simulink model "holo"  (R2012b)
settings: Solver=FixedStepDiscrete  SolverMode=SingleTasking  StartTime=0.0  StopTime=160000  RelTol=1e-3
undefined symbols (not defined in the file): xlipgetpartsetting
libraries: xbsIndex_r4 x3259, casper_library_misc x36, simulink x18, dspsigops x12, casper_library_delays x8, xps_library x5, casper_library_multipliers x4
(part 1 of 34)
settings Model: Creator=Administrator  LastModifiedBy=brains
settings DataIOCC: SignalLoggingSaveFormat=ModelDataLogs
settings OptimizationCC: InitFltsAndDblsToZero=on
settings DebuggingCC: FcnCallInpInsideContextMsg=UseLocalSettings  StrictBusMsg=Warning
settings GRTTargetCC: CombineOutputUpdateFcns=off  GRTInterface=on

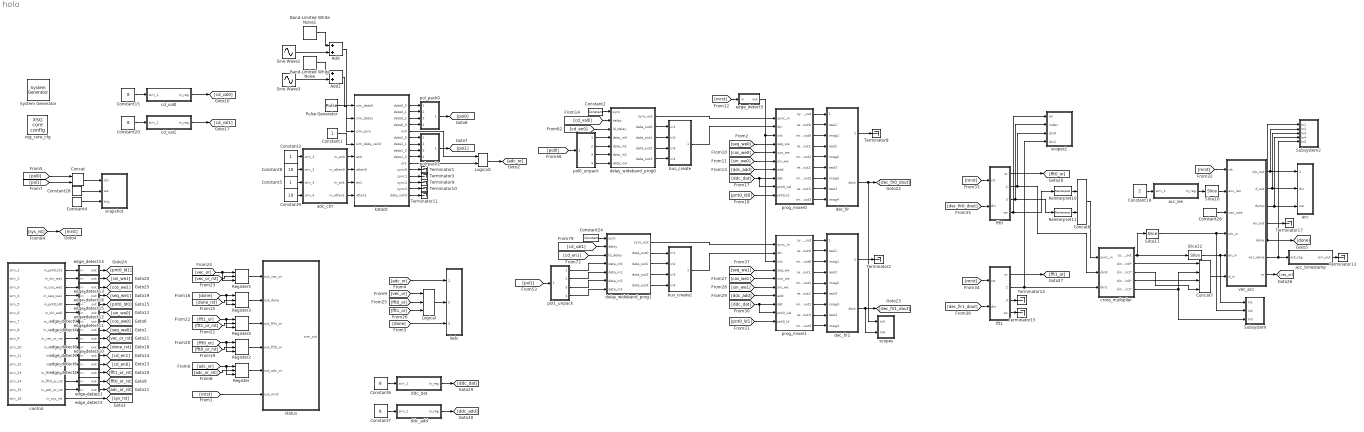
== system holo ==
  " System Generator" : xbsIndex_r4/ System Generator  Tag=genX  xilinxfamily=virtex5  part=xc5vsx95t  speed=-1  package=ff1136  synthesis_tool=XST  clock_wrapper=Clock Enables  directory=./holo/sysgen  proj_type=Project Navigator  Synth_file=XST Defaults  Impl_file=ISE Defaults  testbench=off  simulink_period=1  sysclk_period=5  dcm_input_clock_period=100  incr_netlist=off  trim_vbits=Everywhere in SubSystem  dbl_ovrd=According to Block Masks  core_generation=According to Block Masks  run_coregen=off  deprecated_control=off  eval_field=0  block_type=sysgen
      settings: block_version=10.1.3
  Add : Sum
  Add1 : Sum
  Band-Limited White Noise : simulink/Sources/Band-Limited White Noise  Cov=[0.02]  Ts=0.1  seed=[23341]
  Band-Limited White Noise1 : simulink/Sources/Band-Limited White Noise  Cov=[0.01]  Ts=0.1  seed=[23345]
  Concat : xbsIndex_r4/Concat  num_inputs=2  dbl_ovrd=off  block_type=concat
      settings: block_version=10.1.3
  Concat7 : xbsIndex_r4/Concat  num_inputs=4  dbl_ovrd=off  block_type=concat
      settings: block_version=10.1.3
  Concat8 : xbsIndex_r4/Concat  num_inputs=2  dbl_ovrd=off  block_type=concat
      settings: block_version=10.1.3
  Constant1 : Constant  SampleTime=1/4
  Constant{6..7,15,20} (4 alike) : Constant  Value=8
  Constant19 : Constant  Value=2
  Constant2 : xbsIndex_r4/Constant  const=0  gui_display_data_type=Fixed-point  arith_type=Boolean  n_bits=16  bin_pt=14  preci_type=Single  exp_width=8  frac_width=24  explicit_period=on  period=1  equ=P=C  opselect=C  inp2=PCIN>>17  opr=+  inp1=P  carry=CIN  dbl_ovrd=off  block_type=constant
  Constant24 : xbsIndex_r4/Constant  const=0  gui_display_data_type=Fixed-point  arith_type=Boolean  n_bits=16  bin_pt=14  preci_type=Single  exp_width=8  frac_width=24  explicit_period=on  period=1  equ=P=C  opselect=C  inp2=PCIN>>17  opr=+  inp1=P  carry=CIN  dbl_ovrd=off  block_type=constant
  Constant26 : xbsIndex_r4/Constant  const=4096  gui_display_data_type=Fixed-point  arith_type=Unsigned  n_bits=13  bin_pt=0  preci_type=Single  exp_width=8  frac_width=24  explicit_period=off  period=1  equ=P=C  opselect=C  inp2=PCIN>>17  opr=+  inp1=P  carry=CIN  dbl_ovrd=off  block_type=constant
  Constant28 : xbsIndex_r4/Constant  const=1  gui_display_data_type=Fixed-point  arith_type=Boolean  n_bits=16  bin_pt=14  preci_type=Single  exp_width=8  frac_width=24  explicit_period=off  period=1  equ=P=C  opselect=C  inp2=PCIN>>17  opr=+  inp1=P  carry=CIN  dbl_ovrd=off  block_type=constant
  Constant3 : Constant
  Constant4 : xbsIndex_r4/Constant  const=1  gui_display_data_type=Fixed-point  arith_type=Boolean  n_bits=16  bin_pt=14  preci_type=Single  exp_width=8  frac_width=24  explicit_period=off  period=1  equ=P=C  opselect=C  inp2=PCIN>>17  opr=+  inp1=P  carry=CIN  dbl_ovrd=off  block_type=constant
  Constant5 : Constant
  Constant8 : Constant  Value=10
  Constant9 : Constant  Value=10
  Logical : xbsIndex_r4/Logical  logical_function=OR  inputs=3  en=off  latency=1  precision=Full  arith_type=Unsigned  n_bits=16  bin_pt=0  align_bp=on  dbl_ovrd=off  block_type=logical
  Logical1 : xbsIndex_r4/Logical  logical_function=OR  inputs=2  en=off  latency=1  precision=Full  arith_type=Unsigned  n_bits=16  bin_pt=0  align_bp=on  dbl_ovrd=off  block_type=logical
  Pulse Generator : DiscretePulseGenerator  Period=2^14  PhaseDelay=11  SampleTime=1/4
  Register{,2..5} (5 alike) : xbsIndex_r4/Register  init=0  rst=on  en=on  dbl_ovrd=off  block_type=register
  Reinterpret10 : xbsIndex_r4/Reinterpret  force_arith_type=on  arith_type=Unsigned  force_bin_pt=on  bin_pt=0  block_type=reinterpret
      settings: infoedit="Changes signal type without altering the binary representation.   You can changed the signal between signed and unsigned, and relocate the binary point.<br><br>Hardware notes: In hardware this block costs nothing.<br><br>Example:  Suppose the input is 6 bits wide, signed, with 2 fractional bits, and the output is forced to unsigned with 0 fractional bits.  Then an input of -2.0 (1110.00 in binary 2's complement) becomes an output of 56 (111000 in binary)."
  Reinterpret11 : xbsIndex_r4/Reinterpret  force_arith_type=on  arith_type=Unsigned  force_bin_pt=on  bin_pt=0  block_type=reinterpret
      settings: infoedit="Changes signal type without altering the binary representation.   You can changed the signal between signed and unsigned, and relocate the binary point.<br><br>Hardware notes: In hardware this block costs nothing.<br><br>Example:  Suppose the input is 6 bits wide, signed, with 2 fractional bits, and the output is forced to unsigned with 0 fractional bits.  Then an input of -2.0 (1110.00 in binary 2's complement) becomes an output of 56 (111000 in binary)."
  Sine Wave2 : Sin  Amplitude=0.1  Frequency=57.5/524 * 2 * pi *4  Samples=57.5/524  SampleTime=1/4
  Sine Wave3 : Sin  Amplitude=0.2  Frequency=57.5/524 * 2 * pi *4  Samples=57.5/524  SampleTime=1/4
  Slice10 : xbsIndex_r4/Slice  nbits=16  boolean_output=off  mode=Lower Bit Location + Width  bit1=0  base1=MSB of Input  bit0=0  base0=LSB of Input  dbl_ovrd=off  block_type=slice
      settings: infoedit="Extracts a given range of bits from each input sample and presents it at the output.  The output type is ordinarily unsigned with binary point at zero, but can be Boolean when the slice is one bit wide.<P><P>Hardware notes: In hardware this block costs nothing."  block_version=10.1.3
  Slice11 : xbsIndex_r4/Slice  nbits=12  boolean_output=off  mode=Lower Bit Location + Width  bit1=0  base1=MSB of Input  bit0=0  base0=LSB of Input  dbl_ovrd=off  block_type=slice
      settings: block_version=10.1.3
  Slice12 : xbsIndex_r4/Slice  nbits=1  boolean_output=on  mode=Upper Bit Location + Width  bit1=0  base1=MSB of Input  bit0=0  base0=LSB of Input  dbl_ovrd=off  block_type=slice
      settings: infoedit="Extracts a given range of bits from each input sample and presents it at the output.  The output type is ordinarily unsigned with binary point at zero, but can be Boolean when the slice is one bit wide.<P><P>Hardware notes: In hardware this block costs nothing."  block_version=10.1.3
  Subsystem : Subsystem
  Subsystem2 : Subsystem
  Terminator{1..3,8..11,13..15,17} (11 alike) : Terminator
  acc : Subsystem  mask{bit_width=76, bit_width_o=32, num_chans=12}
      mask prompts: bit_width "Bit width in"; bit_width_o "Bit width out"; num_chans "Number of channels (2^?)"
  acc_len : Subsystem  Tag=xps:sw_reg  AncestorBlock=xps_library/software register  mask(swreg){io_dir=From Processor, io_delay=0, sample_period=1, names=reg, bitwidths=32, bin_pts=0, arith_types=0, sim_port=on, show_format=on}
      mask prompts: io_dir "I/O direction"; io_delay "I/O delay"; sample_period "Sample period"; names "Bitfield names [msb...lsb]"; bitwidths "Bitfield widths"; bin_pts "Bitfield binary pts"; arith_types "Bitfield types, ufix=0, fix=1, bool=2"; sim_port "Provide sim input/output?"; show_format "Print format string?"
      mask help: A 32-bit software-accessible register. Can be divided into bitfields of varying widths and types using the fields in the block mask.
      mask init:
      | swreg_init(gcb)
      settings: AttributesFormatString=1input:uf32.0
      mask TypeOptions io_dir: To Processor | From Processor
      mask Callback io_dir:
      | mask_enables = get_param(gcb, 'MaskEnables');
      | mask_names = get_param(gcb, 'MaskNames');
      | if strcmp(get_param(gcb, 'io_dir'), 'To Processor'),
      |     mask_enables{ismember(mask_names, 'sample_period')} = 'off';
      | else
      |     mask_enables{ismember(mask_names, 'sample_period')} = 'on';
      | end
      | set_param(gcb, 'MaskEnables', mask_enables);
  acc_timestamp : Subsystem  Tag=xps:sw_reg  AncestorBlock=xps_library/software register  mask(swreg){io_dir=To Processor, io_delay=0, sample_period=1, names=reg, bitwidths=32, bin_pts=0, arith_types=0, sim_port=on, show_format=on}
      mask prompts: io_dir "I/O direction"; io_delay "I/O delay"; sample_period "Sample period"; names "Bitfield names [msb...lsb]"; bitwidths "Bitfield widths"; bin_pts "Bitfield binary pts"; arith_types "Bitfield types, ufix=0, fix=1, bool=2"; sim_port "Provide sim input/output?"; show_format "Print format string?"
      mask help: A 32-bit software-accessible register. Can be divided into bitfields of varying widths and types using the fields in the block mask.
      mask init:
      | swreg_init(gcb)
      settings: AttributesFormatString=1output:uf32.0
      mask TypeOptions io_dir: To Processor | From Processor
      mask Callback io_dir:
      | mask_enables = get_param(gcb, 'MaskEnables');
      | mask_names = get_param(gcb, 'MaskNames');
      | if strcmp(get_param(gcb, 'io_dir'), 'To Processor'),
      |     mask_enables{ismember(mask_names, 'sample_period')} = 'off';
      | else
      |     mask_enables{ismember(mask_names, 'sample_period')} = 'on';
      | end
      | set_param(gcb, 'MaskEnables', mask_enables);
  adc_ctrl : Subsystem  Tag=xps:sw_reg  AncestorBlock=xps_library/software register  DataTypeOverride=Double  MinMaxOverflowLogging=ForceOff  mask(swreg){io_dir=From Processor, io_delay=0, sample_period=1, names=[en0 atten0 en1 atten1], bitwidths=[1 6 1 6], bin_pts=[0 0 0 0], arith_types=[2 0 2 0], sim_port=on, show_format=on}
      mask prompts: io_dir "I/O direction"; io_delay "I/O delay"; sample_period "Sample period"; names "Bitfield names [msb...lsb]"; bitwidths "Bitfield widths"; bin_pts "Bitfield binary pts"; arith_types "Bitfield types, ufix=0, fix=1, bool=2"; sim_port "Provide sim input/output?"; show_format "Print format string?"
      mask help: A 32-bit software-accessible register. Can be divided into bitfields of varying widths and types using the fields in the block mask.
      mask init:
      | swreg_init(gcb)
      settings: AttributesFormatString=4 inputs:b,uf6.0,b,uf6.0
      mask TypeOptions io_dir: To Processor | From Processor
      mask Callback io_dir:
      | mask_enables = get_param(gcb, 'MaskEnables');
      | mask_names = get_param(gcb, 'MaskNames');
      | if strcmp(get_param(gcb, 'io_dir'), 'To Processor'),
      |     mask_enables{ismember(mask_names, 'sample_period')} = 'off';
      | else
      |     mask_enables{ismember(mask_names, 'sample_period')} = 'on';
      | end
      | set_param(gcb, 'MaskEnables', mask_enables);
  bus_create : Subsystem  AncestorBlock=casper_library_flow_control/bus_create  mask(bus_create){inputNum=4}
      mask prompts: inputNum "Number of inputs:"
      mask init:
      | bus_create_init(gcb,...
      |     'inputNum', inputNum);
  bus_create1 : Subsystem  AncestorBlock=casper_library_flow_control/bus_create  mask(bus_create){inputNum=4}
      mask prompts: inputNum "Number of inputs:"
      mask init:
      | bus_create_init(gcb,...
      |     'inputNum', inputNum);
  cd_val0 : Subsystem  Tag=xps:sw_reg  AncestorBlock=xps_library/software register  mask(swreg){io_dir=From Processor, io_delay=0, sample_period=1, names=reg, bitwidths=8, bin_pts=0, arith_types=0, sim_port=on, show_format=on}
      mask prompts: io_dir "I/O direction"; io_delay "I/O delay"; sample_period "Sample period"; names "Bitfield names [msb...lsb]"; bitwidths "Bitfield widths"; bin_pts "Bitfield binary pts"; arith_types "Bitfield types, ufix=0, fix=1, bool=2"; sim_port "Provide sim input/output?"; show_format "Print format string?"
      mask help: A 32-bit software-accessible register. Can be divided into bitfields of varying widths and types using the fields in the block mask.
      mask init:
      | swreg_init(gcb)
      settings: AttributesFormatString=1input:uf8.0
      mask TypeOptions io_dir: To Processor | From Processor
      mask Callback io_dir:
      | mask_enables = get_param(gcb, 'MaskEnables');
      | mask_names = get_param(gcb, 'MaskNames');
      | if strcmp(get_param(gcb, 'io_dir'), 'To Processor'),
      |     mask_enables{ismember(mask_names, 'sample_period')} = 'off';
      | else
      |     mask_enables{ismember(mask_names, 'sample_period')} = 'on';
      | end
      | set_param(gcb, 'MaskEnables', mask_enables);
  cd_val1 : Subsystem  Tag=xps:sw_reg  AncestorBlock=xps_library/software register  mask(swreg){io_dir=From Processor, io_delay=0, sample_period=1, names=reg, bitwidths=8, bin_pts=0, arith_types=0, sim_port=on, show_format=on}
      mask prompts: io_dir "I/O direction"; io_delay "I/O delay"; sample_period "Sample period"; names "Bitfield names [msb...lsb]"; bitwidths "Bitfield widths"; bin_pts "Bitfield binary pts"; arith_types "Bitfield types, ufix=0, fix=1, bool=2"; sim_port "Provide sim input/output?"; show_format "Print format string?"
      mask help: A 32-bit software-accessible register. Can be divided into bitfields of varying widths and types using the fields in the block mask.
      mask init:
      | swreg_init(gcb)
      settings: AttributesFormatString=1input:uf8.0
      mask TypeOptions io_dir: To Processor | From Processor
      mask Callback io_dir:
      | mask_enables = get_param(gcb, 'MaskEnables');
      | mask_names = get_param(gcb, 'MaskNames');
      | if strcmp(get_param(gcb, 'io_dir'), 'To Processor'),
      |     mask_enables{ismember(mask_names, 'sample_period')} = 'off';
      | else
      |     mask_enables{ismember(mask_names, 'sample_period')} = 'on';
      | end
      | set_param(gcb, 'MaskEnables', mask_enables);
  control : Subsystem  Tag=xps:sw_reg  AncestorBlock=xps_library/software register  DataTypeOverride=Double  MinMaxOverflowLogging=ForceOff  mask(swreg){io_dir=From Processor, io_delay=0, sample_period=1, names=[pnt0_ld1 sin_we1 cos_we1 seq_we1 pnt0_ld0 sin_we0 cos_we0 seq_we0 vec_or_rst done_rst cd_en1 cd_en0 fft1_or_rst fft0_or_rst adc_or_rst sys_rst], bitwidths=[1 1 1 1 1 1 1 1 1 1 1 1 1 1 1 1], bin_pts=[0 0 0 0 0 0 0 0 0 0 0 0 0 0 0 0], arith_types=[2 2 2 2 2 2 2 2 2 2 2 2 2 2 2 2], sim_port=on, show_format=on}
      mask prompts: io_dir "I/O direction"; io_delay "I/O delay"; sample_period "Sample period"; names "Bitfield names [msb...lsb]"; bitwidths "Bitfield widths"; bin_pts "Bitfield binary pts"; arith_types "Bitfield types, ufix=0, fix=1, bool=2"; sim_port "Provide sim input/output?"; show_format "Print format string?"
      mask help: A 32-bit software-accessible register. Can be divided into bitfields of varying widths and types using the fields in the block mask.
      mask init:
      | swreg_init(gcb)
      settings: AttributesFormatString=16 inputs:b,b,b,b,b,b,b,b,b,b,b,b,b,b,b,b
      mask TypeOptions io_dir: To Processor | From Processor
      mask Callback io_dir:
      | mask_enables = get_param(gcb, 'MaskEnables');
      | mask_names = get_param(gcb, 'MaskNames');
      | if strcmp(get_param(gcb, 'io_dir'), 'To Processor'),
      |     mask_enables{ismember(mask_names, 'sample_period')} = 'off';
      | else
      |     mask_enables{ismember(mask_names, 'sample_period')} = 'on';
      | end
      | set_param(gcb, 'MaskEnables', mask_enables);
  cross_multiplier : Subsystem  AncestorBlock=casper_library/Correlator/cross_multiplier  mask(cross_multiplier){streams=2, aggregation=1, bit_width_in=32, binary_point_in=18, bit_width_out=65, binary_point_out=36, mult_latency=3, add_latency=1, overflow=Saturate, quantisation=Round  (unbiased: even values), conv_latency=1}
      mask prompts: streams "Number input streams"; aggregation "Aggregation per stream"; bit_width_in "Bit width in"; binary_point_in "Binary point in"; bit_width_out "Bit width out"; binary_point_out "Binary point out"; mult_latency "Multiplier latency"; add_latency "Adder latency"; overflow "Overflow behaviour"; quantisation "Quantisation behaviour"; conv_latency "Bit width conversion latency"
      mask help: Cross multiplies aggregated complex input streams.
      mask init:
      | cross_multiplier_init(gcb, ...
      |     'streams', streams, ...
      |     'aggregation', aggregation, ...
      |     'bit_width_in', bit_width_in, ...
      |     'binary_point_in', binary_point_in, ...
      |     'bit_width_out', bit_width_out, ...
      |     'binary_point_out', binary_point_out, ...
      |     'mult_latency', mult_latency, ...
      |     'add_latency', add_latency, ...
      |     'overflow', overflow, ...
      |     'quantisation', quantisation, ...
      |     'conv_latency', conv_latency);
      mask TypeOptions overflow: Wrap | Saturate | Error
      mask TypeOptions quantisation: Truncate | Round  (unbiased: +/- Inf) | Round  (unbiased: even values)
  ddc_add : Subsystem  Tag=xps:sw_reg  AncestorBlock=xps_library/software register  DataTypeOverride=Double  MinMaxOverflowLogging=ForceOff  mask(swreg){io_dir=From Processor, io_delay=0, sample_period=1, names=reg, bitwidths=11, bin_pts=0, arith_types=0, sim_port=on, show_format=on}
      mask prompts: io_dir "I/O direction"; io_delay "I/O delay"; sample_period "Sample period"; names "Bitfield names [msb...lsb]"; bitwidths "Bitfield widths"; bin_pts "Bitfield binary pts"; arith_types "Bitfield types, ufix=0, fix=1, bool=2"; sim_port "Provide sim input/output?"; show_format "Print format string?"
      mask help: A 32-bit software-accessible register. Can be divided into bitfields of varying widths and types using the fields in the block mask.
      mask init:
      | swreg_init(gcb)
      settings: AttributesFormatString=1input:uf11.0
      mask TypeOptions io_dir: To Processor | From Processor
      mask Callback io_dir:
      | mask_enables = get_param(gcb, 'MaskEnables');
      | mask_names = get_param(gcb, 'MaskNames');
      | if strcmp(get_param(gcb, 'io_dir'), 'To Processor'),
      |     mask_enables{ismember(mask_names, 'sample_period')} = 'off';
      | else
      |     mask_enables{ismember(mask_names, 'sample_period')} = 'on';
      | end
      | set_param(gcb, 'MaskEnables', mask_enables);
  ddc_dat : Subsystem  Tag=xps:sw_reg  AncestorBlock=xps_library/software register  mask(swreg){io_dir=From Processor, io_delay=0, sample_period=1, names=reg, bitwidths=32, bin_pts=0, arith_types=0, sim_port=on, show_format=on}
      mask prompts: io_dir "I/O direction"; io_delay "I/O delay"; sample_period "Sample period"; names "Bitfield names [msb...lsb]"; bitwidths "Bitfield widths"; bin_pts "Bitfield binary pts"; arith_types "Bitfield types, ufix=0, fix=1, bool=2"; sim_port "Provide sim input/output?"; show_format "Print format string?"
      mask help: A 32-bit software-accessible register. Can be divided into bitfields of varying widths and types using the fields in the block mask.
      mask init:
      | swreg_init(gcb)
      settings: AttributesFormatString=1input:uf32.0
      mask TypeOptions io_dir: To Processor | From Processor
      mask Callback io_dir:
      | mask_enables = get_param(gcb, 'MaskEnables');
      | mask_names = get_param(gcb, 'MaskNames');
      | if strcmp(get_param(gcb, 'io_dir'), 'To Processor'),
      |     mask_enables{ismember(mask_names, 'sample_period')} = 'off';
      | else
      |     mask_enables{ismember(mask_names, 'sample_period')} = 'on';
      | end
      | set_param(gcb, 'MaskEnables', mask_enables);
  dec_fir : Subsystem  Tag=casper:dec_fir  AncestorBlock=casper_library_downconverter/dec_fir  mask(dec_fir){n_inputs=4, coeff=|, n_bits=25, n_bits_bp=24, quantization=Round  (unbiased: +/- Inf), add_latency=1, mult_latency=2, conv_latency=2, coeff_bit_width=18, coeff_bin_pt=17, absorb_adders=on, adder_imp=Behavioral, lshift=1}
      mask coeff=|
      | [-0.0447689124780572	0.00995075246871881	0.00901304692382896	0.00823242709364412	0.00758382054909261	0.00704464575825092	0.00659455775184286	0.00621523507993219	0.00589020244435913	0.00560468395514498	0.00534548245655601	0.00510088080992406	0.00486056141468576	0.00461554060398477	0.00435811487328397	0.00408181619532124	0.00378137394731173	0.00345268123054543	0.00309276360183094	0.00269974846331496	0.00227283357423222	0.00181225335677420	0.00131924186973398	0.000795991518688312	0.000245606760694299	-0.000327947755040654	-0.000919904991432013	-0.00152475948219077	-0.00213633748961542	-0.00274787324883546	-0.00335209103662813	-0.00394129266271928	-0.00450744985120910	-0.00504230086033329	-0.00553745058111782	-0.00598447326045595	-0.00637501691256493	-0.00670090841536199	-0.00695425823566635	-0.00712756368975998	-0.00721380962406963	-0.00720656539476785	-0.00710007703493642	-0.00688935352347128	-0.00657024611078542	-0.00613951971211587	-0.00559491544916114	-0.00493520350404395	-0.00416022554518398	-0.00327092609143079	-0.00226937229741241	-0.00115876176810638	5.65818574659195e-05	0.00137122567636325	0.00277865662797271	0.00427132277628112	0.00584068646574818	0.00747728890789533	0.00917082561895388	0.0109102319975610	0.0126837782072967	0.0144791724134059	0.0162836713178909	0.0180841968436693	0.0198674577379365	0.0216200747983420	0.0233287083740046	0.0249801867575000	0.0265616340642831	0.0280605961929114	0.0294651634730190	0.0307640886382082	0.0319468988075302	0.0330040002215846	0.0339267745567033	0.0347076657323696	0.0353402562318254	0.0358193320725324	0.0361409356903483	0.0363024061374426	0.0363024061374426	0.0361409356903483	0.0358193320725324	0.0353402562318254	0.0347076657323696	0.0339267745567033	0.0330040002215846	0.0319468988075302	0.0307640886382082	0.0294651634730190	0.0280605961929114	0.0265616340642831	0.0249801867575000	0.0233287083740046	0.0216200747983420	0.0198674577379365	0.0180841968436693	0.0162836713178909	0.0144791724134059	0.0126837782072967	0.0109102319975610	0.00917082561895388	0.00747728890789533	0.00584068646574818	0.00427132277628112	0.00277865662797271	0.00137122567636325	5.65818574659195e-05	-0.00115876176810638	-0.00226937229741241	-0.00327092609143079	-0.00416022554518398	-0.00493520350404395	-0.00559491544916114	-0.00613951971211587	-0.00657024611078542	-0.00688935352347128	-0.00710007703493642	-0.00720656539476785	-0.00721380962406963	-0.00712756368975998	-0.00695425823566635	-0.00670090841536199	-0.00637501691256493	-0.00598447326045595	-0.00553745058111782	-0.00504230086033329	-0.00450744985120910	-0.00394129266271928	-0.00335209103662813	-0.00274787324883546	-0.00213633748961542	-0.00152475948219077	-0.000919904991432013	-0.000327947755040654	0.000245606760694299	0.000795991518688312	0.00131924186973398	0.00181225335677420	0.00227283357423222	0.00269974846331496	0.00309276360183094	0.00345268123054543	0.00378137394731173	0.00408181619532124	0.00435811487328397	0.00461554060398477	0.00486056141468576	0.00510088080992406	0.00534548245655601	0.00560468395514498	0.00589020244435913	0.00621523507993219	0.00659455775184286	0.00704464575825092	0.00758382054909261	0.00823242709364412	0.00901304692382896	0.00995075246871881	-0.0447689124780572
      | ]
      mask prompts: n_inputs "Number of Parallel Streams"; coeff "Coefficients"; n_bits "Bit Width Out"; n_bits_bp "Bin Pt Out"; quantization "Quantization Behavior"; add_latency "Add Latency"; mult_latency "Mult Latency"; conv_latency "Convert latency"; coeff_bit_width "Coefficient bit width"; coeff_bin_pt "Coefficient binary point"; absorb_adders "Absorb adders into DSP slices"; adder_imp "Adder implementation"; lshift "Post adder-tree shift"
      mask help: FIR filter which can handle multiple time samples in parallel and decimates down to 1 time sample. If coefficients are symmetric, will automatically fold before multiplying.
      mask init:
      | dec_fir_init(gcb, ...
      |     'n_inputs', n_inputs, ...
      |     'coeff', coeff, ...
      |     'n_bits', n_bits, ...
      |     'n_bits_bp', n_bits_bp, ...
      |     'quantization', quantization, ...
      |     'add_latency', add_latency, ...
      |     'mult_latency', mult_latency, ...
      |     'conv_latency', conv_latency, ...
      |     'coeff_bit_width', coeff_bit_width, ...
      |     'coeff_bin_pt', coeff_bin_pt, ...
      |     'absorb_adders', absorb_adders, ...
      |     'adder_imp', adder_imp, ...
      |     'lshift', lshift);
      settings: AttributesFormatString=|
      | 160 taps
      | 25_24 r/i
      mask TypeOptions quantization: Truncate | Round  (unbiased: +/- Inf) | Round  (unbiased: Even Values)
      mask TypeOptions adder_imp: Behavioral | Fabric | DSP48
  dec_fir1 : Subsystem  Tag=casper:dec_fir  AncestorBlock=casper_library_downconverter/dec_fir  mask(dec_fir){n_inputs=4, coeff=|, n_bits=25, n_bits_bp=24, quantization=Round  (unbiased: +/- Inf), add_latency=1, mult_latency=2, conv_latency=2, coeff_bit_width=18, coeff_bin_pt=17, absorb_adders=on, adder_imp=Behavioral, lshift=1}
      mask coeff=|
      | [-0.0447689124780572	0.00995075246871881	0.00901304692382896	0.00823242709364412	0.00758382054909261	0.00704464575825092	0.00659455775184286	0.00621523507993219	0.00589020244435913	0.00560468395514498	0.00534548245655601	0.00510088080992406	0.00486056141468576	0.00461554060398477	0.00435811487328397	0.00408181619532124	0.00378137394731173	0.00345268123054543	0.00309276360183094	0.00269974846331496	0.00227283357423222	0.00181225335677420	0.00131924186973398	0.000795991518688312	0.000245606760694299	-0.000327947755040654	-0.000919904991432013	-0.00152475948219077	-0.00213633748961542	-0.00274787324883546	-0.00335209103662813	-0.00394129266271928	-0.00450744985120910	-0.00504230086033329	-0.00553745058111782	-0.00598447326045595	-0.00637501691256493	-0.00670090841536199	-0.00695425823566635	-0.00712756368975998	-0.00721380962406963	-0.00720656539476785	-0.00710007703493642	-0.00688935352347128	-0.00657024611078542	-0.00613951971211587	-0.00559491544916114	-0.00493520350404395	-0.00416022554518398	-0.00327092609143079	-0.00226937229741241	-0.00115876176810638	5.65818574659195e-05	0.00137122567636325	0.00277865662797271	0.00427132277628112	0.00584068646574818	0.00747728890789533	0.00917082561895388	0.0109102319975610	0.0126837782072967	0.0144791724134059	0.0162836713178909	0.0180841968436693	0.0198674577379365	0.0216200747983420	0.0233287083740046	0.0249801867575000	0.0265616340642831	0.0280605961929114	0.0294651634730190	0.0307640886382082	0.0319468988075302	0.0330040002215846	0.0339267745567033	0.0347076657323696	0.0353402562318254	0.0358193320725324	0.0361409356903483	0.0363024061374426	0.0363024061374426	0.0361409356903483	0.0358193320725324	0.0353402562318254	0.0347076657323696	0.0339267745567033	0.0330040002215846	0.0319468988075302	0.0307640886382082	0.0294651634730190	0.0280605961929114	0.0265616340642831	0.0249801867575000	0.0233287083740046	0.0216200747983420	0.0198674577379365	0.0180841968436693	0.0162836713178909	0.0144791724134059	0.0126837782072967	0.0109102319975610	0.00917082561895388	0.00747728890789533	0.00584068646574818	0.00427132277628112	0.00277865662797271	0.00137122567636325	5.65818574659195e-05	-0.00115876176810638	-0.00226937229741241	-0.00327092609143079	-0.00416022554518398	-0.00493520350404395	-0.00559491544916114	-0.00613951971211587	-0.00657024611078542	-0.00688935352347128	-0.00710007703493642	-0.00720656539476785	-0.00721380962406963	-0.00712756368975998	-0.00695425823566635	-0.00670090841536199	-0.00637501691256493	-0.00598447326045595	-0.00553745058111782	-0.00504230086033329	-0.00450744985120910	-0.00394129266271928	-0.00335209103662813	-0.00274787324883546	-0.00213633748961542	-0.00152475948219077	-0.000919904991432013	-0.000327947755040654	0.000245606760694299	0.000795991518688312	0.00131924186973398	0.00181225335677420	0.00227283357423222	0.00269974846331496	0.00309276360183094	0.00345268123054543	0.00378137394731173	0.00408181619532124	0.00435811487328397	0.00461554060398477	0.00486056141468576	0.00510088080992406	0.00534548245655601	0.00560468395514498	0.00589020244435913	0.00621523507993219	0.00659455775184286	0.00704464575825092	0.00758382054909261	0.00823242709364412	0.00901304692382896	0.00995075246871881	-0.0447689124780572
      | ]
      mask prompts: n_inputs "Number of Parallel Streams"; coeff "Coefficients"; n_bits "Bit Width Out"; n_bits_bp "Bin Pt Out"; quantization "Quantization Behavior"; add_latency "Add Latency"; mult_latency "Mult Latency"; conv_latency "Convert latency"; coeff_bit_width "Coefficient bit width"; coeff_bin_pt "Coefficient binary point"; absorb_adders "Absorb adders into DSP slices"; adder_imp "Adder implementation"; lshift "Post adder-tree shift"
      mask help: FIR filter which can handle multiple time samples in parallel and decimates down to 1 time sample. If coefficients are symmetric, will automatically fold before multiplying.
      mask init: same as holo/dec_fir
      settings: AttributesFormatString=|
      | 160 taps
      | 25_24 r/i
      mask TypeOptions quantization: Truncate | Round  (unbiased: +/- Inf) | Round  (unbiased: Even Values)
      mask TypeOptions adder_imp: Behavioral | Fabric | DSP48
  delay_wideband_prog0 : Subsystem  AncestorBlock=casper_library/Delays/delay_wideband_prog  mask(delay_wideband_prog){max_delay=4096, n_inputs_bits=2, bram_latency=2, bram_type=Single Port}
      mask prompts: max_delay "Max Delay (Sample Clks)"; n_inputs_bits "Number of Simultaneous Inputs(2^?)"; bram_latency "BRAM Latency"; bram_type "Select type of BRAM"
      mask init:
      | delay_wideband_prog_init(gcb,...
      |     'max_delay',max_delay,...
      |     'n_inputs_bits',n_inputs_bits,...
      |     'bram_latency',bram_latency,...
      |     'bram_type',bram_type);
      settings: AttributesFormatString=Min Delay=5
      mask TypeOptions bram_type: Single Port | Dual Port
  delay_wideband_prog1 : Subsystem  AncestorBlock=casper_library/Delays/delay_wideband_prog  mask(delay_wideband_prog){max_delay=4096, n_inputs_bits=2, bram_latency=2, bram_type=Single Port}
      mask prompts: max_delay "Max Delay (Sample Clks)"; n_inputs_bits "Number of Simultaneous Inputs(2^?)"; bram_latency "BRAM Latency"; bram_type "Select type of BRAM"
      mask init:
      | delay_wideband_prog_init(gcb,...
      |     'max_delay',max_delay,...
      |     'n_inputs_bits',n_inputs_bits,...
      |     'bram_latency',bram_latency,...
      |     'bram_type',bram_type);
      settings: AttributesFormatString=Min Delay=5
      mask TypeOptions bram_type: Single Port | Dual Port
  edge_detect1 : Subsystem  AncestorBlock=casper_library_misc/edge_detect  mask(edge_detect){edge=Rising, polarity=Active High, x_in=[0 0.08 0.08 0.16 0.16 0.24 0.24 0.32 0.32 0.4], y_in=[-1 -1  1  1  1  1  1  1  1  1], x_out=[0.6 0.68 0.68 0.76 0.76 0.84 0.84 0.92 0.92 1], y_out=[-1 -1  1  1 -1 -1 -1 -1 -1 -1]}
      mask prompts: edge "Edge Type"; polarity "Output Polarity"; x_in "Input X Positions"; y_in "Input Y Positions"; x_out "Output X Positions"; y_out "Output Y Positions"
      mask help: Output is active for one-cycle after each edge of the specified type (i.e. rising, falling or both).
      mask init:
      | edge_detect_init(gcb,...
      |     'edge',edge,...
      |     'polarity',polarity,...
      |     'x_in',x_in,...
      |     'x_out',x_out,...
      |     'y_in',y_in,...
      |     'y_out',y_out);
      | 
      | x_in_num=str2num(getfield(getfield(get_param(gcb,'UserData'),'parameters'),'x_in'));
      | x_out_num=str2num(getfield(getfield(get_param(gcb,'UserData'),'parameters'),'x_out'));
      | y_in_num=str2num(getfield(getfield(get_param(gcb,'UserData'),'parameters'),'y_in'));
      | y_out_num=str2num(getfield(getfield(get_param(gcb,'UserData'),'parameters'),'y_out'));
      settings: AttributesFormatString=|
      | rising edges
      | active high
      mask Help: Output is active for one-cycle after each edge of the specified type (i.e. rising, falling, or both).  Latency is zero.
      mask TypeOptions edge: Rising | Falling | Both
      mask TypeOptions polarity: Active High | Active Low
      mask Display:
      | plot(x_in_num,0.5+y_in_num*0.2);
      | plot(x_out_num,0.5+y_out_num*0.2);
  edge_detect10 : Subsystem  AncestorBlock=casper_library_misc/edge_detect  mask(edge_detect){edge=Rising, polarity=Active High, x_in=[0 0.08 0.08 0.16 0.16 0.24 0.24 0.32 0.32 0.4], y_in=[-1 -1  1  1  1  1  1  1  1  1], x_out=[0.6 0.68 0.68 0.76 0.76 0.84 0.84 0.92 0.92 1], y_out=[-1 -1  1  1 -1 -1 -1 -1 -1 -1]}
      mask prompts: edge "Edge Type"; polarity "Output Polarity"; x_in "Input X Positions"; y_in "Input Y Positions"; x_out "Output X Positions"; y_out "Output Y Positions"
      mask help: Output is active for one-cycle after each edge of the specified type (i.e. rising, falling or both).
      mask init: same as holo/edge_detect1
      settings: AttributesFormatString=|
      | rising edges
      | active high
      mask Help: Output is active for one-cycle after each edge of the specified type (i.e. rising, falling, or both).  Latency is zero.
      mask TypeOptions edge: Rising | Falling | Both
      mask TypeOptions polarity: Active High | Active Low
      mask Display:
      | plot(x_in_num,0.5+y_in_num*0.2);
      | plot(x_out_num,0.5+y_out_num*0.2);
  edge_detect11 : Subsystem  AncestorBlock=casper_library_misc/edge_detect  mask(edge_detect){edge=Rising, polarity=Active High, x_in=[0 0.08 0.08 0.16 0.16 0.24 0.24 0.32 0.32 0.4], y_in=[-1 -1  1  1  1  1  1  1  1  1], x_out=[0.6 0.68 0.68 0.76 0.76 0.84 0.84 0.92 0.92 1], y_out=[-1 -1  1  1 -1 -1 -1 -1 -1 -1]}
      mask prompts: edge "Edge Type"; polarity "Output Polarity"; x_in "Input X Positions"; y_in "Input Y Positions"; x_out "Output X Positions"; y_out "Output Y Positions"
      mask help: Output is active for one-cycle after each edge of the specified type (i.e. rising, falling or both).
      mask init: same as holo/edge_detect1
      settings: AttributesFormatString=|
      | rising edges
      | active high
      mask Help: Output is active for one-cycle after each edge of the specified type (i.e. rising, falling, or both).  Latency is zero.
      mask TypeOptions edge: Rising | Falling | Both
      mask TypeOptions polarity: Active High | Active Low
      mask Display:
      | plot(x_in_num,0.5+y_in_num*0.2);
      | plot(x_out_num,0.5+y_out_num*0.2);
  edge_detect12 : Subsystem  AncestorBlock=casper_library_misc/edge_detect  mask(edge_detect){edge=Rising, polarity=Active High, x_in=[0 0.08 0.08 0.16 0.16 0.24 0.24 0.32 0.32 0.4], y_in=[-1 -1  1  1  1  1  1  1  1  1], x_out=[0.6 0.68 0.68 0.76 0.76 0.84 0.84 0.92 0.92 1], y_out=[-1 -1  1  1 -1 -1 -1 -1 -1 -1]}
      mask prompts: edge "Edge Type"; polarity "Output Polarity"; x_in "Input X Positions"; y_in "Input Y Positions"; x_out "Output X Positions"; y_out "Output Y Positions"
      mask help: Output is active for one-cycle after each edge of the specified type (i.e. rising, falling or both).
      mask init: same as holo/edge_detect1
      settings: AttributesFormatString=|
      | rising edges
      | active high
      mask Help: Output is active for one-cycle after each edge of the specified type (i.e. rising, falling, or both).  Latency is zero.
      mask TypeOptions edge: Rising | Falling | Both
      mask TypeOptions polarity: Active High | Active Low
      mask Display:
      | plot(x_in_num,0.5+y_in_num*0.2);
      | plot(x_out_num,0.5+y_out_num*0.2);
  edge_detect13 : Subsystem  AncestorBlock=casper_library_misc/edge_detect  mask(edge_detect){edge=Rising, polarity=Active High, x_in=[0 0.08 0.08 0.16 0.16 0.24 0.24 0.32 0.32 0.4], y_in=[-1 -1  1  1  1  1  1  1  1  1], x_out=[0.6 0.68 0.68 0.76 0.76 0.84 0.84 0.92 0.92 1], y_out=[-1 -1  1  1 -1 -1 -1 -1 -1 -1]}
      mask prompts: edge "Edge Type"; polarity "Output Polarity"; x_in "Input X Positions"; y_in "Input Y Positions"; x_out "Output X Positions"; y_out "Output Y Positions"
      mask help: Output is active for one-cycle after each edge of the specified type (i.e. rising, falling or both).
      mask init: same as holo/edge_detect1
      settings: AttributesFormatString=|
      | rising edges
      | active high
      mask Help: Output is active for one-cycle after each edge of the specified type (i.e. rising, falling, or both).  Latency is zero.
      mask TypeOptions edge: Rising | Falling | Both
      mask TypeOptions polarity: Active High | Active Low
      mask Display:
      | plot(x_in_num,0.5+y_in_num*0.2);
      | plot(x_out_num,0.5+y_out_num*0.2);
  edge_detect14 : Subsystem  AncestorBlock=casper_library_misc/edge_detect  mask(edge_detect){edge=Rising, polarity=Active High, x_in=[0 0.08 0.08 0.16 0.16 0.24 0.24 0.32 0.32 0.4], y_in=[-1 -1  1  1  1  1  1  1  1  1], x_out=[0.6 0.68 0.68 0.76 0.76 0.84 0.84 0.92 0.92 1], y_out=[-1 -1  1  1 -1 -1 -1 -1 -1 -1]}
      mask prompts: edge "Edge Type"; polarity "Output Polarity"; x_in "Input X Positions"; y_in "Input Y Positions"; x_out "Output X Positions"; y_out "Output Y Positions"
      mask help: Output is active for one-cycle after each edge of the specified type (i.e. rising, falling or both).
      mask init: same as holo/edge_detect1
      settings: AttributesFormatString=|
      | rising edges
      | active high
      mask Help: Output is active for one-cycle after each edge of the specified type (i.e. rising, falling, or both).  Latency is zero.
      mask TypeOptions edge: Rising | Falling | Both
      mask TypeOptions polarity: Active High | Active Low
      mask Display:
      | plot(x_in_num,0.5+y_in_num*0.2);
      | plot(x_out_num,0.5+y_out_num*0.2);
  edge_detect15 : Subsystem  AncestorBlock=casper_library_misc/edge_detect  mask(edge_detect){edge=Rising, polarity=Active High, x_in=[0 0.08 0.08 0.16 0.16 0.24 0.24 0.32 0.32 0.4], y_in=[-1 -1  1  1  1  1  1  1  1  1], x_out=[0.6 0.68 0.68 0.76 0.76 0.84 0.84 0.92 0.92 1], y_out=[-1 -1  1  1 -1 -1 -1 -1 -1 -1]}
      mask prompts: edge "Edge Type"; polarity "Output Polarity"; x_in "Input X Positions"; y_in "Input Y Positions"; x_out "Output X Positions"; y_out "Output Y Positions"
      mask help: Output is active for one-cycle after each edge of the specified type (i.e. rising, falling or both).
      mask init: same as holo/edge_detect1
      settings: AttributesFormatString=|
      | rising edges
      | active high
      mask Help: Output is active for one-cycle after each edge of the specified type (i.e. rising, falling, or both).  Latency is zero.
      mask TypeOptions edge: Rising | Falling | Both
      mask TypeOptions polarity: Active High | Active Low
      mask Display:
      | plot(x_in_num,0.5+y_in_num*0.2);
      | plot(x_out_num,0.5+y_out_num*0.2);
  edge_detect16 : Subsystem  AncestorBlock=casper_library_misc/edge_detect  mask(edge_detect){edge=Rising, polarity=Active High, x_in=[0 0.08 0.08 0.16 0.16 0.24 0.24 0.32 0.32 0.4], y_in=[-1 -1  1  1  1  1  1  1  1  1], x_out=[0.6 0.68 0.68 0.76 0.76 0.84 0.84 0.92 0.92 1], y_out=[-1 -1  1  1 -1 -1 -1 -1 -1 -1]}
      mask prompts: edge "Edge Type"; polarity "Output Polarity"; x_in "Input X Positions"; y_in "Input Y Positions"; x_out "Output X Positions"; y_out "Output Y Positions"
      mask help: Output is active for one-cycle after each edge of the specified type (i.e. rising, falling or both).
      mask init: same as holo/edge_detect1
      settings: AttributesFormatString=|
      | rising edges
      | active high
      mask Help: Output is active for one-cycle after each edge of the specified type (i.e. rising, falling, or both).  Latency is zero.
      mask TypeOptions edge: Rising | Falling | Both
      mask TypeOptions polarity: Active High | Active Low
      mask Display:
      | plot(x_in_num,0.5+y_in_num*0.2);
      | plot(x_out_num,0.5+y_out_num*0.2);
  edge_detect2 : Subsystem  AncestorBlock=casper_library_misc/edge_detect  mask(edge_detect){edge=Rising, polarity=Active High, x_in=[0 0.08 0.08 0.16 0.16 0.24 0.24 0.32 0.32 0.4], y_in=[-1 -1  1  1  1  1  1  1  1  1], x_out=[0.6 0.68 0.68 0.76 0.76 0.84 0.84 0.92 0.92 1], y_out=[-1 -1  1  1 -1 -1 -1 -1 -1 -1]}
      mask prompts: edge "Edge Type"; polarity "Output Polarity"; x_in "Input X Positions"; y_in "Input Y Positions"; x_out "Output X Positions"; y_out "Output Y Positions"
      mask help: Output is active for one-cycle after each edge of the specified type (i.e. rising, falling or both).
      mask init: same as holo/edge_detect1
      settings: AttributesFormatString=|
      | rising edges
      | active high
      mask Help: Output is active for one-cycle after each edge of the specified type (i.e. rising, falling, or both).  Latency is zero.
      mask TypeOptions edge: Rising | Falling | Both
      mask TypeOptions polarity: Active High | Active Low
      mask Display:
      | plot(x_in_num,0.5+y_in_num*0.2);
      | plot(x_out_num,0.5+y_out_num*0.2);
  edge_detect3 : Subsystem  AncestorBlock=casper_library_misc/edge_detect  mask(edge_detect){edge=Rising, polarity=Active High, x_in=[0 0.08 0.08 0.16 0.16 0.24 0.24 0.32 0.32 0.4], y_in=[-1 -1  1  1  1  1  1  1  1  1], x_out=[0.6 0.68 0.68 0.76 0.76 0.84 0.84 0.92 0.92 1], y_out=[-1 -1  1  1 -1 -1 -1 -1 -1 -1]}
      mask prompts: edge "Edge Type"; polarity "Output Polarity"; x_in "Input X Positions"; y_in "Input Y Positions"; x_out "Output X Positions"; y_out "Output Y Positions"
      mask help: Output is active for one-cycle after each edge of the specified type (i.e. rising, falling or both).
      mask init: same as holo/edge_detect1
      settings: AttributesFormatString=|
      | rising edges
      | active high
      mask Help: Output is active for one-cycle after each edge of the specified type (i.e. rising, falling, or both).  Latency is zero.
      mask TypeOptions edge: Rising | Falling | Both
      mask TypeOptions polarity: Active High | Active Low
      mask Display:
      | plot(x_in_num,0.5+y_in_num*0.2);
      | plot(x_out_num,0.5+y_out_num*0.2);
  edge_detect4 : Subsystem  AncestorBlock=casper_library_misc/edge_detect  mask(edge_detect){edge=Rising, polarity=Active High, x_in=[0 0.08 0.08 0.16 0.16 0.24 0.24 0.32 0.32 0.4], y_in=[-1 -1  1  1  1  1  1  1  1  1], x_out=[0.6 0.68 0.68 0.76 0.76 0.84 0.84 0.92 0.92 1], y_out=[-1 -1  1  1 -1 -1 -1 -1 -1 -1]}
      mask prompts: edge "Edge Type"; polarity "Output Polarity"; x_in "Input X Positions"; y_in "Input Y Positions"; x_out "Output X Positions"; y_out "Output Y Positions"
      mask help: Output is active for one-cycle after each edge of the specified type (i.e. rising, falling or both).
      mask init: same as holo/edge_detect1
      settings: AttributesFormatString=|
      | rising edges
      | active high
      mask Help: Output is active for one-cycle after each edge of the specified type (i.e. rising, falling, or both).  Latency is zero.
      mask TypeOptions edge: Rising | Falling | Both
      mask TypeOptions polarity: Active High | Active Low
      mask Display:
      | plot(x_in_num,0.5+y_in_num*0.2);
      | plot(x_out_num,0.5+y_out_num*0.2);
  edge_detect5 : Subsystem  AncestorBlock=casper_library/Misc/edge_detect  mask(edge_detect){edge=Falling, polarity=Active High, x_in=[0 0.08 0.08 0.16 0.16 0.24 0.24 0.32 0.32 0.4], y_in=[1  1 -1 -1 -1 -1 -1 -1 -1 -1], x_out=[0.6 0.68 0.68 0.76 0.76 0.84 0.84 0.92 0.92 1], y_out=[-1 -1  1  1 -1 -1 -1 -1 -1 -1]}
      mask prompts: edge "Edge Type"; polarity "Output Polarity"; x_in "Input X Positions"; y_in "Input Y Positions"; x_out "Output X Positions"; y_out "Output Y Positions"
      mask help: Output is active for one-cycle after each edge of the specified type (i.e. rising, falling or both).
      mask init: same as holo/edge_detect1
      settings: AttributesFormatString=|
      | falling edges
      | active high
      mask Help: Output is active for one-cycle after each edge of the specified type (i.e. rising, falling, or both).  Latency is zero.
      mask TypeOptions edge: Rising | Falling | Both
      mask TypeOptions polarity: Active High | Active Low
      mask Display:
      | plot(x_in_num,0.5+y_in_num*0.2);
      | plot(x_out_num,0.5+y_out_num*0.2);
  edge_detect6 : Subsystem  AncestorBlock=casper_library_misc/edge_detect  mask(edge_detect){edge=Rising, polarity=Active High, x_in=[0 0.08 0.08 0.16 0.16 0.24 0.24 0.32 0.32 0.4], y_in=[-1 -1  1  1  1  1  1  1  1  1], x_out=[0.6 0.68 0.68 0.76 0.76 0.84 0.84 0.92 0.92 1], y_out=[-1 -1  1  1 -1 -1 -1 -1 -1 -1]}
      mask prompts: edge "Edge Type"; polarity "Output Polarity"; x_in "Input X Positions"; y_in "Input Y Positions"; x_out "Output X Positions"; y_out "Output Y Positions"
      mask help: Output is active for one-cycle after each edge of the specified type (i.e. rising, falling or both).
      mask init: same as holo/edge_detect1
      settings: AttributesFormatString=|
      | rising edges
      | active high
      mask Help: Output is active for one-cycle after each edge of the specified type (i.e. rising, falling, or both).  Latency is zero.
      mask TypeOptions edge: Rising | Falling | Both
      mask TypeOptions polarity: Active High | Active Low
      mask Display:
      | plot(x_in_num,0.5+y_in_num*0.2);
      | plot(x_out_num,0.5+y_out_num*0.2);
  edge_detect7 : Subsystem  AncestorBlock=casper_library_misc/edge_detect  mask(edge_detect){edge=Rising, polarity=Active High, x_in=[0 0.08 0.08 0.16 0.16 0.24 0.24 0.32 0.32 0.4], y_in=[-1 -1  1  1  1  1  1  1  1  1], x_out=[0.6 0.68 0.68 0.76 0.76 0.84 0.84 0.92 0.92 1], y_out=[-1 -1  1  1 -1 -1 -1 -1 -1 -1]}
      mask prompts: edge "Edge Type"; polarity "Output Polarity"; x_in "Input X Positions"; y_in "Input Y Positions"; x_out "Output X Positions"; y_out "Output Y Positions"
      mask help: Output is active for one-cycle after each edge of the specified type (i.e. rising, falling or both).
      mask init: same as holo/edge_detect1
      settings: AttributesFormatString=|
      | rising edges
      | active high
      mask Help: Output is active for one-cycle after each edge of the specified type (i.e. rising, falling, or both).  Latency is zero.
      mask TypeOptions edge: Rising | Falling | Both
      mask TypeOptions polarity: Active High | Active Low
      mask Display:
      | plot(x_in_num,0.5+y_in_num*0.2);
      | plot(x_out_num,0.5+y_out_num*0.2);
  edge_detect8 : Subsystem  AncestorBlock=casper_library_misc/edge_detect  mask(edge_detect){edge=Rising, polarity=Active High, x_in=[0 0.08 0.08 0.16 0.16 0.24 0.24 0.32 0.32 0.4], y_in=[-1 -1  1  1  1  1  1  1  1  1], x_out=[0.6 0.68 0.68 0.76 0.76 0.84 0.84 0.92 0.92 1], y_out=[-1 -1  1  1 -1 -1 -1 -1 -1 -1]}
      mask prompts: edge "Edge Type"; polarity "Output Polarity"; x_in "Input X Positions"; y_in "Input Y Positions"; x_out "Output X Positions"; y_out "Output Y Positions"
      mask help: Output is active for one-cycle after each edge of the specified type (i.e. rising, falling or both).
      mask init: same as holo/edge_detect1
      settings: AttributesFormatString=|
      | rising edges
      | active high
      mask Help: Output is active for one-cycle after each edge of the specified type (i.e. rising, falling, or both).  Latency is zero.
      mask TypeOptions edge: Rising | Falling | Both
      mask TypeOptions polarity: Active High | Active Low
      mask Display:
      | plot(x_in_num,0.5+y_in_num*0.2);
      | plot(x_out_num,0.5+y_out_num*0.2);
  edge_detect9 : Subsystem  AncestorBlock=casper_library_misc/edge_detect  mask(edge_detect){edge=Rising, polarity=Active High, x_in=[0 0.08 0.08 0.16 0.16 0.24 0.24 0.32 0.32 0.4], y_in=[-1 -1  1  1  1  1  1  1  1  1], x_out=[0.6 0.68 0.68 0.76 0.76 0.84 0.84 0.92 0.92 1], y_out=[-1 -1  1  1 -1 -1 -1 -1 -1 -1]}
      mask prompts: edge "Edge Type"; polarity "Output Polarity"; x_in "Input X Positions"; y_in "Input Y Positions"; x_out "Output X Positions"; y_out "Output Y Positions"
      mask help: Output is active for one-cycle after each edge of the specified type (i.e. rising, falling or both).
      mask init: same as holo/edge_detect1
      settings: AttributesFormatString=|
      | rising edges
      | active high
      mask Help: Output is active for one-cycle after each edge of the specified type (i.e. rising, falling, or both).  Latency is zero.
      mask TypeOptions edge: Rising | Falling | Both
      mask TypeOptions polarity: Active High | Active Low
      mask Display:
      | plot(x_in_num,0.5+y_in_num*0.2);
      | plot(x_out_num,0.5+y_out_num*0.2);
  fft0 : Subsystem  mask{din_bit_width=25, din_bin_pt=24, dout_bit_width=32, fft_chans=12}
      mask prompts: din_bit_width "Input data width"; din_bin_pt "input data binary point"; dout_bit_width "Output data width"; fft_chans "Channels in FFT (2^?)"
      mask init:
      | bit_growth = fft_chans+1;
      | allowance = dout_bit_width-din_bit_width;
      | dout_bin_pt = min(din_bin_pt, din_bin_pt - (bit_growth-allowance));
      | set_param([gcb,'/convert_of0'], ...
      |     'bit_width_i', tostring(din_bit_width+fft_chans+1), ...
      |     'binary_point_i', tostring(din_bin_pt), ...
      |     'bit_width_o', tostring(dout_bit_width), ...
      |     'binary_point_o', tostring(dout_bin_pt));
      | set_param([gcb,'/convert_of1'], ...
      |     'bit_width_i', tostring(din_bit_width+fft_chans+1), ...
      |     'binary_point_i', tostring(din_bin_pt), ...
      |     'bit_width_o', tostring(dout_bit_width), ...
      |     'binary_point_o', tostring(dout_bin_pt));
      | set_param([gcb,'/fft'], ...
      |     'transform_length', tostring(2^fft_chans));
      | set_param([gcb,'/fifo'], ...
      |     'depth', [num2str(2^fft_chans/1024),'K']);
  fft1 : Subsystem  mask{din_bit_width=25, din_bin_pt=24, dout_bit_width=32, fft_chans=12}
      mask prompts: din_bit_width "Input data width"; din_bin_pt "input data binary point"; dout_bit_width "Output data width"; fft_chans "Channels in FFT (2^?)"
      mask init: same as holo/fft0
  katadc : Subsystem  Tag=xps:katadc  AncestorBlock=xps_library/katadc  mask(katadc){adc_brd=adc0, adc_interleave=off, bypass_auto=off, en_gain=on, adc_clk_rate=132*4, sample_period=1}
      mask prompts: adc_brd "ADC board"; adc_interleave "ADC interleave mode"; bypass_auto "Bypass auto config"; en_gain "Enable gain"; adc_clk_rate "ADC sampling rate (MHz)"; sample_period "Sample period"
      mask init:
      | name = gcb;
      | katadc_init(gcb, ...
      |     'name', name, ...
      |     'adc_brd', adc_brd, ...
      |     'adc_interleave', adc_interleave, ...
      |     'bypass_auto', bypass_auto, ...
      |     'en_gain', en_gain, ...
      |     'adc_clk_rate', adc_clk_rate, ...
      |     'sample_period', sample_period);
      mask TypeOptions adc_brd: adc0 | adc1
  leds : Subsystem
  pol0_unpack : Subsystem
  pol1_unpack : Subsystem
  pol_pack0 : Subsystem
  pol_pack1 : Subsystem
  prog_mixer0 : Subsystem  AncestorBlock=holo_library/Downconverter/prog_mixer  mask{lookup_bits=9, coeff_bits=25, streams=4, din_bits=8, add_latency=1, bram_latency=2, mult_latency=2, numerator=28, denominator=262, offset=0, dout_bits=24, dout_bin_pt=23}
      mask prompts: lookup_bits "Lookup depth (2^?)"; coeff_bits "Coefficient resolution (bits)"; din_bits "Input data resolution (bits)"; add_latency "Adder latency"; bram_latency "BRAM latency"; mult_latency "Multiplier latency"; numerator "Numerator of preloaded frequency (N in N/Mxsampling frequency)"; denominator "Denominator of preloaded frequency (M in N/Mxsampling frequency)"; offset "Initial phase offset"; dout_bits "Output data bit width"; dout_bin_pt "Output data binary point"
  prog_mixer1 : Subsystem  AncestorBlock=holo_library/Downconverter/prog_mixer  mask{lookup_bits=9, coeff_bits=25, streams=4, din_bits=8, add_latency=1, bram_latency=2, mult_latency=2, numerator=28, denominator=262, offset=0, dout_bits=24, dout_bin_pt=23}
      mask prompts: lookup_bits "Lookup depth (2^?)"; coeff_bits "Coefficient resolution (bits)"; din_bits "Input data resolution (bits)"; add_latency "Adder latency"; bram_latency "BRAM latency"; mult_latency "Multiplier latency"; numerator "Numerator of preloaded frequency (N in N/Mxsampling frequency)"; denominator "Denominator of preloaded frequency (M in N/Mxsampling frequency)"; offset "Initial phase offset"; dout_bits "Output data bit width"; dout_bin_pt "Output data binary point"
  scopes : Subsystem
  scopes1 : Subsystem
  snapshot : Subsystem  Tag=casper:snapshot  AncestorBlock=casper_library_scopes/snapshot  mask(snapshot){storage=bram, dram_dimm=1, dram_clock=200, nsamples=10, data_width=64, offset=off, circap=off, value=off, use_dsp48=on}
      mask prompts: storage "Storage medium"; dram_dimm "DRAM dimm"; dram_clock "DRAM clock rate"; nsamples "Number of Samples (2^?)"; data_width "Data width"; offset "Start delay support"; circap "Circular capture support"; value "Extra value capture support"; use_dsp48 "Use DSP48s to implement counters"
      mask help:
      | Standard snap block, but with the following optional extras;
      |  1) Optionally delay the fabric trigger by a user-specified number of valids.
      |  2) Capture continuously after a trigger until a stop pulse is received. Data is captured into BRAM continuously, with old data being overwritten until a stop command is received. Then stop capturing when memory is filled. This enables you to get some data before and some data after the stop pulse. Use the 'tr_en_cnt' register to determine where you are in your vector. 'Addr' register's MSb now indicates 'busy capturing'.
      |  3) Optionally capture a value on an input port to a register at the same time as the first data sample.
      |  4) Implement counters using DSP48Es to save resources.
      mask init:
      | snapshot_init(gcb, ...
      |     'storage', storage, ...
      |     'dram_dimm', dram_dimm, ...
      |     'dram_clock', dram_clock, ...
      |     'nsamples', nsamples, ...
      |     'data_width', data_width, ...
      |     'offset', offset, ...
      |     'circap', circap, ...
      |     'value', value, ...
      |     'use_dsp48', use_dsp48);
      mask TypeOptions storage: bram | dram
      mask Callback storage: snapshot_callback();
      mask TypeOptions dram_dimm: 1 | 2 | 3 | 4
      mask TypeOptions dram_clock: 200 | 250 | 266 | 300 | 333
      mask TypeOptions data_width: 8 | 16 | 32 | 64 | 128
  status : Subsystem  Tag=xps:sw_reg  AncestorBlock=xps_library/software register  DataTypeOverride=Double  MinMaxOverflowLogging=ForceOff  mask(swreg){io_dir=To Processor, io_delay=0, sample_period=1, names=[vec_or done fft1_or fft0_or adc_or mrst], bitwidths=[1 1 1 1 1 1], bin_pts=[0 0 0 0 0 0], arith_types=[2 2 2 2 2 2], sim_port=on, show_format=on}
      mask prompts: io_dir "I/O direction"; io_delay "I/O delay"; sample_period "Sample period"; names "Bitfield names [msb...lsb]"; bitwidths "Bitfield widths"; bin_pts "Bitfield binary pts"; arith_types "Bitfield types, ufix=0, fix=1, bool=2"; sim_port "Provide sim input/output?"; show_format "Print format string?"
      mask help: A 32-bit software-accessible register. Can be divided into bitfields of varying widths and types using the fields in the block mask.
      mask init:
      | swreg_init(gcb)
      settings: AttributesFormatString=6 outputs:b,b,b,b,b,b
      mask TypeOptions io_dir: To Processor | From Processor
      mask Callback io_dir:
      | mask_enables = get_param(gcb, 'MaskEnables');
      | mask_names = get_param(gcb, 'MaskNames');
      | if strcmp(get_param(gcb, 'io_dir'), 'To Processor'),
      |     mask_enables{ismember(mask_names, 'sample_period')} = 'off';
      | else
      |     mask_enables{ismember(mask_names, 'sample_period')} = 'on';
      | end
      | set_param(gcb, 'MaskEnables', mask_enables);
  vec_acc : Subsystem  mask{inputs=4, din_bits=65, din_bin_pt=36, acc_width=76, vec_bits=12, acc_bits=16, bram_latency=2, add_latency=2}
      mask prompts: inputs "Input streams"; din_bits "Input data width (bits)"; din_bin_pt "Input data binary point"; acc_width "Accumulator width (bits)"; vec_bits "Maximum vector size (2^?)"; acc_bits "Maximum accumulations (2^?)"; bram_latency "BRAM latency"; add_latency "Adder latency"
      mask init:
      | set_param([gcb,'/add'], ...
      |     'din_bits', tostring(din_bits), ...
      |     'din_bin_pt', tostring(din_bin_pt), ...
      |     'acc_bits', tostring(acc_width));
  xsg_core_cfg : xps_library/XSG core config  Tag=xps:xsg  hw_sys=ROACH:sx95t  clk_src=adc0_clk  ROACH_clk_src=adc0_clk  ROACH2_clk_src=sys_clk  MKDIG_clk_src=sys_clk  clk_rate=200  sample_period=1  synthesis_tool=XST
  wires:
  [sys_rst] -> [mrst]
  pol_pack1/1(Out1) -> [pol1]
  pol_pack0/1(Out1) -> [pol0]
  Pulse Generator/1 -> katadc/3(sim_sync)
  Constant1/1 -> katadc/4(sim_data_valid)
  Constant4/1 -> snapshot/3(trig)
  edge_detect3/1(out) -> [adc_or_rst]
  [adc_or] -> Register/1, Register/3
  [adc_or_rst] -> Register/2
  [pol0] -> pol0_unpack/1(In1)
  [pol1] -> pol1_unpack/1(In1)
  [cd_val0] -> delay_wideband_prog0/2(delay)
  [cd_val1] -> delay_wideband_prog1/2(delay)
  [cd_en1] -> delay_wideband_prog1/3(ld_delay)
  pol1_unpack/1(Out1) -> delay_wideband_prog1/4(data_in0)
  pol1_unpack/2(Out2) -> delay_wideband_prog1/5(data_in1)
  pol1_unpack/3(Out3) -> delay_wideband_prog1/6(data_in2)
  pol1_unpack/4(Out4) -> delay_wideband_prog1/7(data_in3)
  delay_wideband_prog0/1(sync_out) -> prog_mixer0/1(sync_in)
  prog_mixer0/1(sync_out) -> dec_fir/1(sync_in)
  prog_mixer0/2(real_out0) -> dec_fir/2(real1)
  prog_mixer0/3(imag_out0) -> dec_fir/3(imag1)
  prog_mixer0/4(real_out1) -> dec_fir/4(real2)
  prog_mixer0/5(imag_out1) -> dec_fir/5(imag2)
  prog_mixer0/6(real_out2) -> dec_fir/6(real3)
  prog_mixer0/7(imag_out2) -> dec_fir/7(imag3)
  prog_mixer0/8(real_out3) -> dec_fir/8(real4)
  prog_mixer0/9(imag_out3) -> dec_fir/9(imag4)
  [mrst] -> edge_detect5/1(in)
  edge_detect5/1(out) -> prog_mixer0/3(init), prog_mixer1/3(init)
  delay_wideband_prog1/1(sync_out) -> prog_mixer1/1(sync_in)
  prog_mixer1/1(sync_out) -> dec_fir1/1(sync_in)
  prog_mixer1/2(real_out0) -> dec_fir1/2(real1)
  prog_mixer1/3(imag_out0) -> dec_fir1/3(imag1)
  prog_mixer1/4(real_out1) -> dec_fir1/4(real2)
  prog_mixer1/5(imag_out1) -> dec_fir1/5(imag2)
  prog_mixer1/6(real_out2) -> dec_fir1/6(real3)
  prog_mixer1/7(imag_out2) -> dec_fir1/7(imag3)
  prog_mixer1/8(real_out3) -> dec_fir1/8(real4)
  prog_mixer1/9(imag_out3) -> dec_fir1/9(imag4)
  dec_fir1/1(sync_out) -> Terminator2/1
  edge_detect6/1(out) -> [cd_en0]
  edge_detect7/1(out) -> [cd_en1]
  cd_val0/1(in_reg) -> [cd_val0]
  cd_val1/1(in_reg) -> [cd_val1]
  dec_fir1/2(dout) -> scopes/2(In6), [dec_fir1_dout]
  edge_detect8/1(out) -> [done_rst]
  [done] -> Register3/1, Register3/3
  [done_rst] -> Register3/2
  Constant2/1 -> delay_wideband_prog0/1(sync)
  Constant24/1 -> delay_wideband_prog1/1(sync)
  dec_fir/1(sync_out) -> Terminator8/1
  Concat/1 -> snapshot/1(din)
  Constant28/1 -> snapshot/2(we)
  [pol0] -> Concat/1
  [pol1] -> Concat/2
  [fft0_or] -> Register2/1, Register2/3
  [fft0_or_rst] -> Register2/2
  edge_detect1/1(out) -> [fft0_or_rst]
  edge_detect2/1(out) -> [fft1_or_rst]
  [fft1_or] -> Register4/3, Register4/1
  [fft1_or_rst] -> Register4/2
  edge_detect10/1(out) -> [vec_or_rst]
  [vec_or] -> Register5/3, Register5/1
  [vec_or_rst] -> Register5/2
  [adc_or] -> leds/1(adc_or)
  [vec_or] -> Logical/1
  [fft0_or] -> Logical/2
  [fft1_or] -> Logical/3
  fft0/2(dout) -> scopes1/3(din0), cross_multiplier/2(din0)
  fft0/3(index) -> scopes1/2(index), Reinterpret11/1
  fft0/4(en) -> scopes1/1(en), Reinterpret10/1
  Concat8/1 -> cross_multiplier/1(sync_in)
  cross_multiplier/5(din1_x_din1*) -> Concat7/2, Subsystem/3(In3)
  Reinterpret10/1 -> Concat8/1
  Reinterpret11/1 -> Concat8/2
  cross_multiplier/1(sync_out) -> Slice12/1, Slice11/1
  Constant19/1 -> acc_len/1(sim_1)
  acc_len/1(in_reg) -> Slice10/1
  fft1/2(dout) -> scopes1/4(din1), cross_multiplier/3(din1)
  fft1/3(index) -> Terminator14/1
  fft1/4(en) -> Terminator15/1
  vec_acc/4(en_out) -> Terminator17/1
  vec_acc/5(done) -> [done], Subsystem2/1(In1)
  vec_acc/6(acc_done) -> Subsystem2/5(In5), acc_timestamp/1(out_reg)
  Concat7/1 -> vec_acc/6(d_in)
  Slice12/1 -> vec_acc/5(en_in), Subsystem/1(In1)
  Slice11/1 -> vec_acc/4(idx_in), Subsystem/2(In2)
  Slice10/1 -> vec_acc/2(acc_len)
  [mrst] -> vec_acc/1(rst)
  vec_acc/1(idx_out) -> Subsystem2/2(In2), acc/1(index)
  vec_acc/2(d_out) -> Subsystem2/3(In3), acc/2(din)
  cross_multiplier/2(din0_x_din0*) -> Concat7/1
  vec_acc/3(dump) -> acc/3(we), Subsystem2/4(In4)
  fft1/1(or) -> [fft1_or]
  fft0/1(or) -> [fft0_or]
  Constant26/1 -> vec_acc/3(vec_size)
  acc_timestamp/1(sim_out) -> Terminator13/1
  vec_acc/7(or) -> [vec_or]
  [mrst] -> fft0/1(rst)
  [dec_fir0_dout] -> fft0/2(din)
  [mrst] -> fft1/1(rst)
  [dec_fir1_dout] -> fft1/2(din)
  Register5/1 -> status/1(out_vec_or)
  Register3/1 -> status/2(out_done)
  Register4/1 -> status/3(out_fft1_or)
  Register2/1 -> status/4(out_fft0_or)
  Register/1 -> status/5(out_adc_or)
  [mrst] -> status/6(out_mrst)
  Logical1/1 -> [adc_or]
  katadc/1(data0_0) -> pol_pack0/1(In1)
  katadc/2(data0_1) -> pol_pack0/2(In2)
  katadc/3(data0_2) -> pol_pack0/3(In3)
  katadc/4(data0_3) -> pol_pack0/4(In4)
  katadc/10(or1) -> Logical1/2
  katadc/11(sync0) -> Terminator1/1
  katadc/12(sync1) -> Terminator3/1
  katadc/13(sync2) -> Terminator9/1
  katadc/14(sync3) -> Terminator10/1
  katadc/15(data_valid) -> Terminator11/1
  Logical/1 -> leds/2(dsp_or)
  [done] -> leds/3(done)
  Sine Wave2/1 -> Add/2
  Sine Wave3/1 -> Add1/2
  Add1/1 -> katadc/2(sim_data1)
  Add/1 -> katadc/1(sim_data0)
  Band-Limited White Noise1/1 -> Add/1
  Band-Limited White Noise/1 -> Add1/1
  dec_fir/2(dout) -> [dec_fir0_dout], scopes/1(In5)
  edge_detect4/1(out) -> [seq_we0]
  edge_detect9/1(out) -> [cos_we0]
  edge_detect11/1(out) -> [sin_we0]
  edge_detect12/1(out) -> [pnt0_ld0]
  edge_detect15/1(out) -> [seq_we1]
  edge_detect16/1(out) -> [cos_we1]
  edge_detect13/1(out) -> [sin_we1]
  edge_detect14/1(out) -> [pnt0_ld1]
  Constant6/1 -> ddc_dat/1(sim_1)
  Constant7/1 -> ddc_add/1(sim_1)
  ddc_add/1(in_reg) -> [ddc_add]
  [seq_we0] -> prog_mixer0/4(seq_we)
  [cos_we0] -> prog_mixer0/5(cos_we)
  [sin_we0] -> prog_mixer0/6(sin_we)
  [ddc_add] -> prog_mixer0/7(add)
  [ddc_dat] -> prog_mixer0/8(dat), prog_mixer0/9(pnt0_val)
  [pnt0_ld0] -> prog_mixer0/10(pnt0_ld)
  [seq_we1] -> prog_mixer1/4(seq_we)
  [cos_we1] -> prog_mixer1/5(cos_we)
  [sin_we1] -> prog_mixer1/6(sin_we)
  [ddc_add] -> prog_mixer1/7(add)
  [ddc_dat] -> prog_mixer1/9(pnt0_val), prog_mixer1/8(dat)
  [pnt0_ld1] -> prog_mixer1/10(pnt0_ld)
  [cd_en0] -> delay_wideband_prog0/3(ld_delay)
  pol0_unpack/1(Out1) -> delay_wideband_prog0/4(data_in0)
  pol0_unpack/2(Out2) -> delay_wideband_prog0/5(data_in1)
  pol0_unpack/3(Out3) -> delay_wideband_prog0/6(data_in2)
  pol0_unpack/4(Out4) -> delay_wideband_prog0/7(data_in3)
  katadc/5(or0) -> Logical1/1
  katadc/6(data1_0) -> pol_pack1/1(In1)
  katadc/7(data1_1) -> pol_pack1/2(In2)
  katadc/8(data1_2) -> pol_pack1/3(In3)
  katadc/9(data1_3) -> pol_pack1/4(In4)
  control/16(in_sys_rst) -> [sys_rst]
  control/15(in_adc_or_rst) -> edge_detect3/1(in)
  control/14(in_fft0_or_rst) -> edge_detect1/1(in)
  control/13(in_fft1_or_rst) -> edge_detect2/1(in)
  control/12(in_cd_en0) -> edge_detect6/1(in)
  control/11(in_cd_en1) -> edge_detect7/1(in)
  control/10(in_done_rst) -> edge_detect8/1(in)
  control/9(in_vec_or_rst) -> edge_detect10/1(in)
  control/8(in_seq_we0) -> edge_detect4/1(in)
  control/7(in_cos_we0) -> edge_detect9/1(in)
  control/6(in_sin_we0) -> edge_detect11/1(in)
  control/5(in_pnt0_ld0) -> edge_detect12/1(in)
  control/4(in_seq_we1) -> edge_detect15/1(in)
  control/3(in_cos_we1) -> edge_detect16/1(in)
  control/2(in_sin_we1) -> edge_detect13/1(in)
  control/1(in_pnt0_ld1) -> edge_detect14/1(in)
  ddc_dat/1(in_reg) -> [ddc_dat]
  Constant15/1 -> cd_val0/1(sim_1)
  adc_ctrl/4(in_atten1) -> katadc/8(atten1)
  adc_ctrl/3(in_en1) -> katadc/7(en1)
  adc_ctrl/2(in_atten0) -> katadc/6(atten0)
  adc_ctrl/1(in_en0) -> katadc/5(en0)
  Constant3/1 -> adc_ctrl/1(sim_1)
  Constant5/1 -> adc_ctrl/3(sim_3)
  Constant9/1 -> adc_ctrl/4(sim_4)
  Constant8/1 -> adc_ctrl/2(sim_2)
  delay_wideband_prog0/5(data_out3) -> bus_create/4(in4)
  delay_wideband_prog0/4(data_out2) -> bus_create/3(in3)
  delay_wideband_prog0/3(data_out1) -> bus_create/2(in2)
  delay_wideband_prog0/2(data_out0) -> bus_create/1(in1)
  bus_create/1(bus_out) -> prog_mixer0/2(din)
  delay_wideband_prog1/2(data_out0) -> bus_create1/1(in1)
  delay_wideband_prog1/3(data_out1) -> bus_create1/2(in2)
  delay_wideband_prog1/4(data_out2) -> bus_create1/3(in3)
  delay_wideband_prog1/5(data_out3) -> bus_create1/4(in4)
  bus_create1/1(bus_out) -> prog_mixer1/2(din)
  Constant20/1 -> cd_val1/1(sim_1)
  cross_multiplier/3(din0_x_din1*) -> Concat7/3
  cross_multiplier/4(din1_x_din0*) -> Concat7/4
